simulink model "Simulink_Navigation_block"  (R2016b)
settings: Solver=VariableStepAuto  StartTime=0.0  StopTime=10.0  RelTol=1e-3
values from neighbouring files (symbols this model uses):
  Xgeodetic = [lat0;lon0;h0]    [initial.m]
settings Model: Creator=asus  LastModifiedBy=osx

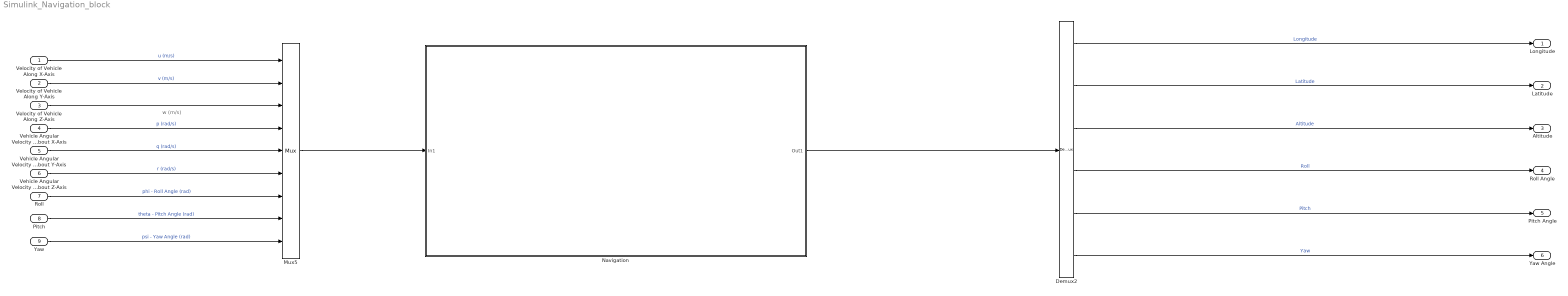
== system Simulink_Navigation_block ==
  note: w (m/s)
  Velocity of Vehicle Along X-Axis : Inport
  Velocity of Vehicle Along Y-Axis : Inport  Port=2
  Velocity of Vehicle Along Z-Axis : Inport  Port=3
  Vehicle Angular Velocity About X-Axis : Inport  Port=4
  Vehicle Angular Velocity About Y-Axis : Inport  Port=5
  Vehicle Angular Velocity About Z-Axis : Inport  Port=6
  Roll : Inport  Port=7
  Pitch : Inport  Port=8
  Yaw : Inport  Port=9
  Demux2 : Demux  Outputs=6
  Mux5 : Mux  Inputs=9
  Navigation : Subsystem  Description=|
      | Author: Reza Samarghandi
      | 
      | Email: RezaSamarghandi@yahoo.com
  Longitude : Outport
  Latitude : Outport  Port=2
  Altitude : Outport  Port=3
  Roll Angle : Outport  Port=4
  Pitch Angle : Outport  Port=5
  Yaw Angle : Outport  Port=6
  wires:
  Demux2/1 -> Longitude/1  "Longitude"
  Demux2/2 -> Latitude/1  "Latitude"
  Demux2/3 -> Altitude/1  "Altitude"
  Demux2/4 -> Roll Angle/1  "Roll"
  Demux2/5 -> Pitch Angle/1  "Pitch"
  Demux2/6 -> Yaw Angle/1  "Yaw"
  Roll/1 -> Mux5/7  "phi - Roll Angle (rad)"
  Pitch/1 -> Mux5/8  "theta - Pitch Angle (rad)"
  Yaw/1 -> Mux5/9  "psi - Yaw Angle (rad)"
  Velocity of Vehicle Along X-Axis/1 -> Mux5/1  "u (m/s)"
  Velocity of Vehicle Along Y-Axis/1 -> Mux5/2  "v (m/s)"
  Velocity of Vehicle Along Z-Axis/1 -> Mux5/3
  Vehicle Angular Velocity About X-Axis/1 -> Mux5/4  "p (rad/s)"
  Vehicle Angular Velocity About Y-Axis/1 -> Mux5/5  "q (rad/s)"
  Vehicle Angular Velocity About Z-Axis/1 -> Mux5/6  "r (rad/s)"
  Mux5/1 -> Navigation/1(In1)
  Navigation/1(Out1) -> Demux2/1

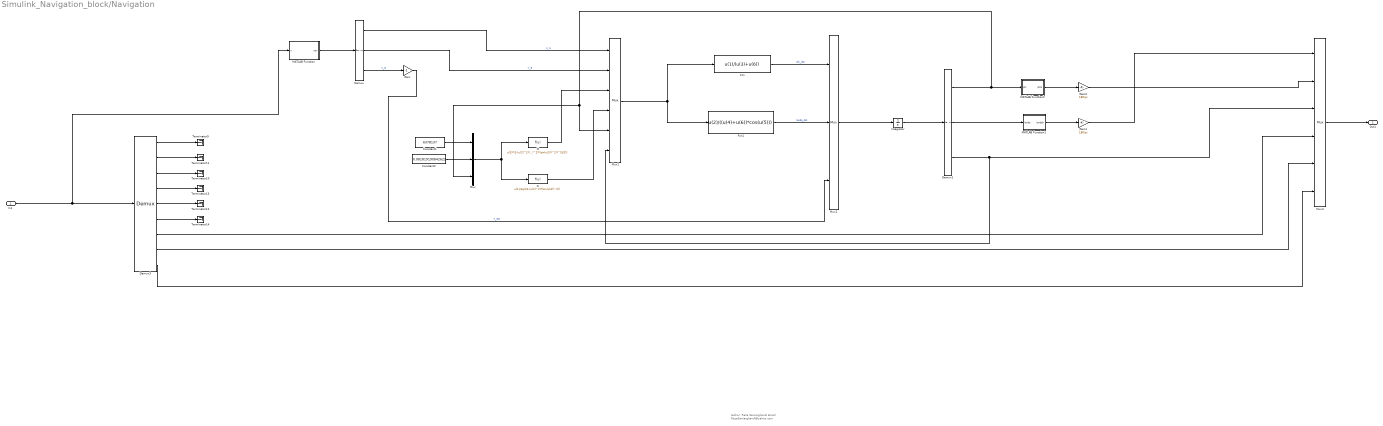
== system Simulink_Navigation_block/Navigation ==
  note: Author: Reza Samarghandi
      |
      | Email: RezaSamarghandi@yahoo.com
  In1 : Inport
  Constant1 : Constant  Value=6378137
  Constant2 : Constant  Value=0.081819190842622
  Demux : Demux  Outputs=3
  Demux1 : Demux  Outputs=3
  Demux3 : Demux  Outputs=9
  Fcn : Fcn  Expr=u(1)/(u(3)+u(6))
  Fcn1 : Fcn  Expr=u(2)/((u(4)+u(6))*cos(u(5)))
  Gain : Gain  Gain=-1
  Gain1 : Gain  Gain=180/pi
  Gain2 : Gain  Gain=180/pi
  Integrator : Integrator  InitialCondition=Xgeodetic
  M : Fcn  Expr=u(1)*(1-(u(2)^2))/((1-(u(2)^2)*(sin(u(3))^2))^(3/2))
  MATLAB Function : MATLAB Function  TreatAsAtomicUnit=on
  MATLAB Function1 : MATLAB Function  TreatAsAtomicUnit=on
  MATLAB Function2 : MATLAB Function  TreatAsAtomicUnit=on
  Mux : Mux  Inputs=3
  Mux1 : Mux  Inputs=6
  Mux2 : Mux  Inputs=3
  Mux3 : Mux  Inputs=6
  N : Fcn  Expr=u(1)/sqrt(1-(u(2)^2)*(sin(u(3))^2))
  Terminator{9..14} (6 alike) : Terminator
  Out1 : Outport
  wires:
  MATLAB Function/1(nav) -> Demux/1
  Demux/3 -> Gain/1  "V_D"
  Demux/2 -> Mux1/2  "V_E"
  Demux1/3 -> Mux3/3, Mux1/6
  Demux3/5 -> Terminator12/1
  In1/1 -> MATLAB Function/1(u), Demux3/1
  MATLAB Function2/1(phib) -> Gain2/1
  N/1 -> Mux1/4
  Integrator/1 -> Demux1/1
  Demux3/9 -> Mux3/6
  Mux/1 -> N/1, M/1
  Mux1/1 -> Fcn1/1, Fcn/1
  Demux3/4 -> Terminator13/1
  MATLAB Function1/1(landab) -> Gain1/1
  Fcn1/1 -> Mux2/2  "landa_dot"
  Demux3/1 -> Terminator9/1
  Demux1/1 -> MATLAB Function2/1(phi), Mux1/5, Mux/3
  Mux2/1 -> Integrator/1
  Mux3/1 -> Out1/1
  Demux3/6 -> Terminator14/1
  Gain1/1 -> Mux3/1
  Constant2/1 -> Mux/2
  Demux3/8 -> Mux3/5
  Demux/1 -> Mux1/1  "V_N"
  Gain2/1 -> Mux3/2
  Demux3/7 -> Mux3/4
  Constant1/1 -> Mux/1
  Gain/1 -> Mux2/3  "h_dot"
  Demux1/2 -> MATLAB Function1/1(landa)
  Demux3/3 -> Terminator10/1
  Demux3/2 -> Terminator11/1
  Fcn/1 -> Mux2/1  "phi_dot"
  M/1 -> Mux1/3

== matlab function Simulink_Navigation_block/Navigation/MATLAB Function1 ==
  data: landa input; landab output
function landab =landabound(landa)

if landa>(pi)
    landab= landa-2*pi;
elseif landa<(-pi)
    landab=landa+2*pi;
else
    landab=landa;
end
landab;

== matlab function Simulink_Navigation_block/Navigation/MATLAB Function ==
  data: u input; nav output
function nav =navigation(u)


v=u(1:3);
an=u(7:9);

V_b=[v(1); v(2); v(3)];

phi=an(1);
theta=an(2);
psi=an(3);

c1v=[cos(psi), sin(psi), 0;
     -sin(psi), cos(psi), 0;
     0, 0, 1];
 
 c21=[cos(theta), 0, -sin(theta);
      0, 1, 0;
      sin(theta), 0, cos(theta)];
  
 cb2=[1, 0, 0;
      0, cos(phi), sin(phi);
      0, -sin(phi), cos(phi)];
  
 cbv=cb2*c21*c1v;
 cvb=cbv';
 
 nav=cvb*V_b;

== matlab function Simulink_Navigation_block/Navigation/MATLAB Function2 ==
  data: phi input; phib output
function phib =phibound(phi)

if phi>(pi/2)
    phib= phi-pi;
elseif phi<(-pi/2)
    phib=phi+pi;
else
    phib=phi;
end
phib;
